simulink model "SS_task8_2_2020"  (R2020b)
settings: Solver=VariableStepAuto  StartTime=0.0  StopTime=10.0  RelTol=1e-3
values from neighbouring files (symbols this model uses):
  A_ss_2dof_vh = eval(subs(A_ss_2dof_vh_sym,{c1,c2},[c,c]))    [Copy_of_Lab_3_ale.m]    (also in Lab_3_ale.m; SS_task9.m = [0 1 0 0; out8_2.mat = [0 -54.5454545455 0 0 1 -3.63636363636 0 0 0 0 0 -61.7142857; out9.mat = [0 -54.5454545455 0 0 1 0 0 0 0 0 0 -61.7142857143 ... (16 e)
  B_ss_2dof_vh = eval(subs(B_ss_2dof_vh_sym,{c1,c2},[c,c]))    [Copy_of_Lab_3_ale.m]    (also in Lab_3_ale.m; SS_task9.m = [0 0 0 0; out8_2.mat = [0 27.2727272727 0 -163.636363636 0 1.81818181818 0 -0.34285; out9.mat = [0 27.2727272727 0 -5.14285714286 0 27.2727272727 0 5.142857)
  C_ss_2dof_vh = [1 0 0 0 ... (first row only)    [Copy_of_Lab_3_ale.m]    (also in Lab_3_ale.m; SS_task9.m = [0 1 0 0; out8_2.mat = [1  0  0  0; 0  0  1  0]; out9.mat = [0  1  0  0; 0  0  0  1])
  D_ss_2dof_vh = [0 0 0 0; 0 0 0 0]    [Copy_of_Lab_3_ale.m]    (also in Lab_3_ale.m; SS_task9.m = [0 0 0 0; out8_2.mat = [0  0  0  0; 0  0  0  0]; out9.mat = [0  0  0  0; 0  0  0  0])
undefined symbols (not defined in the file or in its folder): sigbuilder_block
settings Model: Creator=rivaa  LastModifiedBy=rivaa
settings DebuggingCC: SFMachineParentedDataDiag=error

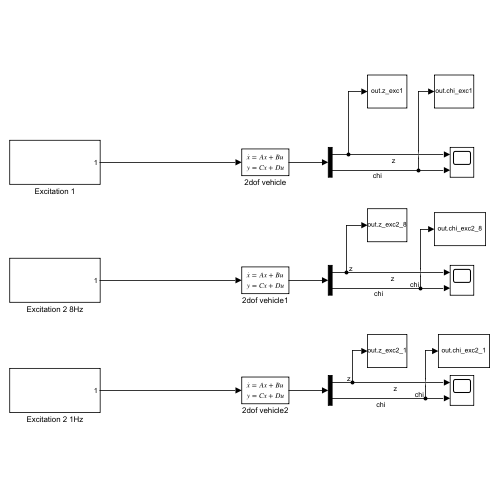
[thumbnail: Simulink's stored preview of the top-level diagram]
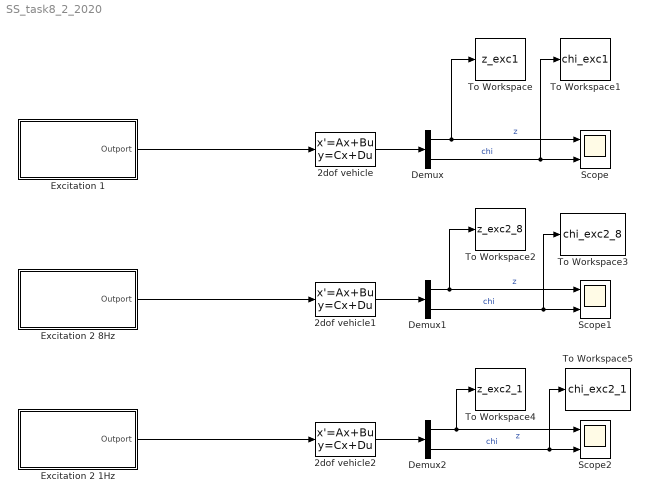
== system SS_task8_2_2020 ==
  2dof vehicle : StateSpace  A=A_ss_2dof_vh  B=B_ss_2dof_vh  C=C_ss_2dof_vh  D=D_ss_2dof_vh  InitialCondition=0
  2dof vehicle1 : StateSpace  A=A_ss_2dof_vh  B=B_ss_2dof_vh  C=C_ss_2dof_vh  D=D_ss_2dof_vh  InitialCondition=0
  2dof vehicle2 : StateSpace  A=A_ss_2dof_vh  B=B_ss_2dof_vh  C=C_ss_2dof_vh  D=D_ss_2dof_vh  InitialCondition=0
  Demux : Demux  Outputs=2
  Demux1 : Demux  Outputs=2
  Demux2 : Demux  Outputs=2
  Excitation 1 : Subsystem
  Excitation 2 1Hz : Subsystem
  Excitation 2 8Hz : Subsystem
  Scope : Scope  NumInputPorts=2
  Scope1 : Scope  NumInputPorts=2
  Scope2 : Scope  NumInputPorts=2
  To Workspace : ToWorkspace  VariableName=z_exc1  SampleTime=-1
      settings: Save2DSignal=2-D array (concatenate along first dimension)
  To Workspace1 : ToWorkspace  VariableName=chi_exc1  SampleTime=-1
      settings: Save2DSignal=2-D array (concatenate along first dimension)
  To Workspace2 : ToWorkspace  VariableName=z_exc2_8  SampleTime=-1
      settings: Save2DSignal=2-D array (concatenate along first dimension)
  To Workspace3 : ToWorkspace  VariableName=chi_exc2_8  SampleTime=-1
      settings: Save2DSignal=2-D array (concatenate along first dimension)
  To Workspace4 : ToWorkspace  VariableName=z_exc2_1  SampleTime=-1
      settings: Save2DSignal=2-D array (concatenate along first dimension)
  To Workspace5 : ToWorkspace  VariableName=chi_exc2_1  SampleTime=-1
      settings: Save2DSignal=2-D array (concatenate along first dimension)
  wires:
  Excitation 1/1(Outport) -> 2dof vehicle/1
  2dof vehicle/1 -> Demux/1
  Demux/1 -> Scope/1, To Workspace/1  "z"
  Demux/2 -> To Workspace1/1, Scope/2  "chi"
  2dof vehicle1/1 -> Demux1/1
  Excitation 2 8Hz/1(Outport) -> 2dof vehicle1/1
  2dof vehicle2/1 -> Demux2/1
  Excitation 2 1Hz/1(Outport) -> 2dof vehicle2/1
  Demux1/2 -> To Workspace3/1, Scope1/2  "chi"
  Demux1/1 -> To Workspace2/1, Scope1/1  "z"
  Demux2/1 -> To Workspace4/1, Scope2/1  "z"
  Demux2/2 -> To Workspace5/1, Scope2/2  "chi"

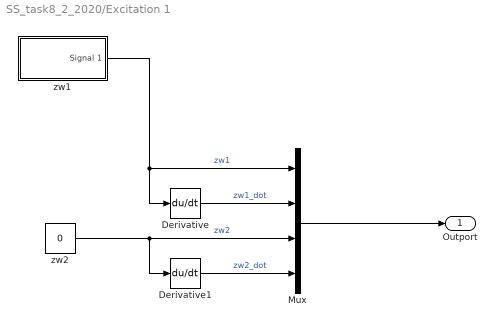
== system SS_task8_2_2020/Excitation 1 ==
  Derivative : Derivative  CoefficientInTFapproximation=0.01
  Derivative1 : Derivative
  Mux : Mux
  zw1 : Subsystem  Tag=STV Subsys  LoadFcn=sigbuilder_block('load');  StartFcn=sigbuilder_block('start');  StopFcn=sigbuilder_block('stop');  ClipboardFcn=sigbuilder_block('clipboard');  mask(Sigbuilder block){tuvar=[0:10]}
      mask help: Simulink:masks:SigbuilderBlock_MD
      mask init:
      | if ~strcmp(get_param(bdroot(gcbh),'SimulationStatus'),'stopped') tuvar = sigbuilder_block('maskInit'); end
      settings: CopyFcn=sigbuilder_block('copy');  DeleteFcn=sigbuilder_block('delete');  ModelCloseFcn=sigbuilder_block('modelClose');  PreSaveFcn=sigbuilder_block('preSave');  PauseFcn=sigbuilder_block('pause');  ContinueFcn=sigbuilder_block('continue');  NameChangeFcn=sigbuilder_block('namechange');  OpenFcn=sigbuilder_block('open',[437.6 199.2 550.4 400 ]);  CloseFcn=sigbuilder_block('close');
      mask Display: plot(0, 0, 100, 100,[2, 2, 32, 32, 2], [68, 8, 8, 68, 68],[32, 2], [38, 38], [32, 19, 2],[53, 60, 44], [32, 17, 17, 2],[16, 16, 31, 31]);txt = getActiveGroup(gcbh);text(2, 100, txt,'verticalAlignment', 'top');
  zw2 : Constant  Value=0
  Outport : Outport
  wires:
  zw1/1(Signal 1) -> Derivative/1, Mux/1  "zw1"
  Mux/1 -> Outport/1
  Derivative/1 -> Mux/2  "zw1_dot"
  zw2/1 -> Derivative1/1, Mux/3  "zw2"
  Derivative1/1 -> Mux/4  "zw2_dot"

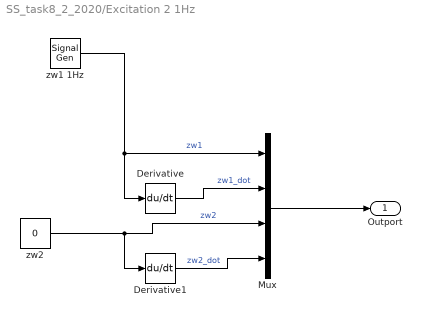
== system SS_task8_2_2020/Excitation 2 1Hz ==
  Derivative : Derivative
  Derivative1 : Derivative
  Mux : Mux
  zw1 1Hz : SignalGenerator  Amplitude=0.01  Frequency=2*pi*1  Units=rad/sec
  zw2 : Constant  Value=0
  Outport : Outport
  wires:
  zw2/1 -> Derivative1/1, Mux/3  "zw2"
  Derivative1/1 -> Mux/4  "zw2_dot"
  zw1 1Hz/1 -> Derivative/1, Mux/1  "zw1"
  Derivative/1 -> Mux/2  "zw1_dot"
  Mux/1 -> Outport/1

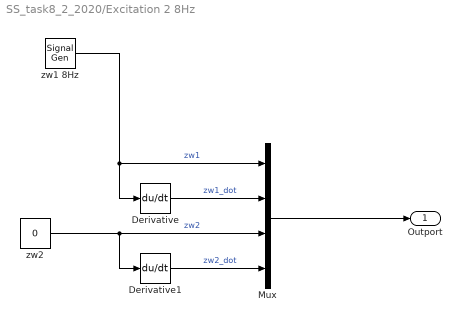
== system SS_task8_2_2020/Excitation 2 8Hz ==
  Derivative : Derivative
  Derivative1 : Derivative
  Mux : Mux
  zw1 8Hz : SignalGenerator  Amplitude=0.01  Frequency=2*pi*8  Units=rad/sec
  zw2 : Constant  Value=0
  Outport : Outport
  wires:
  zw2/1 -> Derivative1/1, Mux/3  "zw2"
  Derivative1/1 -> Mux/4  "zw2_dot"
  zw1 8Hz/1 -> Derivative/1, Mux/1  "zw1"
  Derivative/1 -> Mux/2  "zw1_dot"
  Mux/1 -> Outport/1

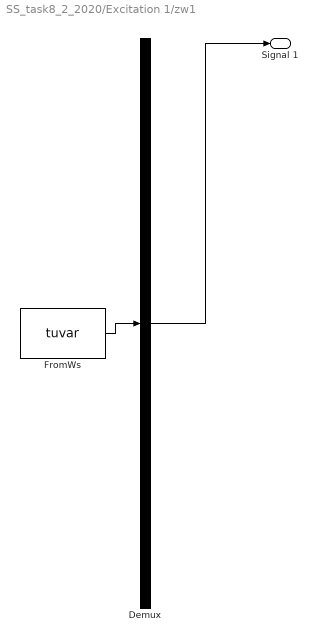
== system SS_task8_2_2020/Excitation 1/zw1 ==
  Demux : Demux  Tag=STV Demux  Outputs=1
      settings: DisplayOption=none
  FromWs : FromWorkspace  Tag=STV FromWs  VariableName=tuvar
      SigBuilderData=|
      | common.afterFinalStr = 'Extrapolate'
      | common.sampleTime = 0
      | dataSet.timeRange = [0 10]
      | dataSet.name = 'Group 1'
      | sbobj.Groups.Name = 'Group 1'
      | sbobj.Groups.Signals.Name = 'Signal 1'
      | sbobj.Groups.Signals.XData = [0 0.1 0.1 10]
      | sbobj.Groups.Signals.YData = [0.03 0.03 0 0]
  Signal 1 : Outport  Tag=STV Outport
  wires:
  Demux/1 -> Signal 1/1
  FromWs/1 -> Demux/1
